simulink model "Glide_slope_controller_d"  (R2019b)
settings: Solver=VariableStepAuto  StartTime=0.0  StopTime=300  RelTol=1e-3
values from neighbouring files (symbols this model uses):
  A_gs = A_longitude_lo([1 3 4 2 5], [1 3 4 2 5])    [FindF16Dynamics.m]    (also in FindF16Dynamics_Chapter8.m)
  alpha = 8.49    [FindF16Dynamics.m]    (also in FindF16Dynamics_Chapter8.m = 10.4511; FindF16Dynamics_KIllian.m; trim_F16.m = alpha*pi/180)
  B_gs = A_longitude_lo([1 3 4 2 5], [6, 7])    [FindF16Dynamics.m]    (also in FindF16Dynamics_Chapter8.m)
  C_gs = C_longitude_lo([1 3 4 2 5], [1 3 4 2 5])    [FindF16Dynamics.m]    (also in FindF16Dynamics_Chapter8.m)
  D_gs = D_longitude_lo([1 3 4 2 5], [1])    [FindF16Dynamics.m]    (also in FindF16Dynamics_Chapter8.m = D_longitude_lo([1 3 4 2 5], [1, 2]))
  thrust = 5000    [FindF16Dynamics.m]    (also in FindF16Dynamics_Chapter8.m = 2826.8165; FindF16Dynamics_KIllian.m)
  velocity = 300    [FindF16Dynamics.m]    (also in FindF16Dynamics_Chapter8.m; FindF16Dynamics_KIllian.m = input('Enter the velocity for the simulation (ft/s):  '); FindF16Dynamics_Q6,7.m = 900; FindF16Dynamics_Q6-7.m = 900)
libraries: simulink x4
settings Model: Creator=tomas  LastModifiedBy=tomas

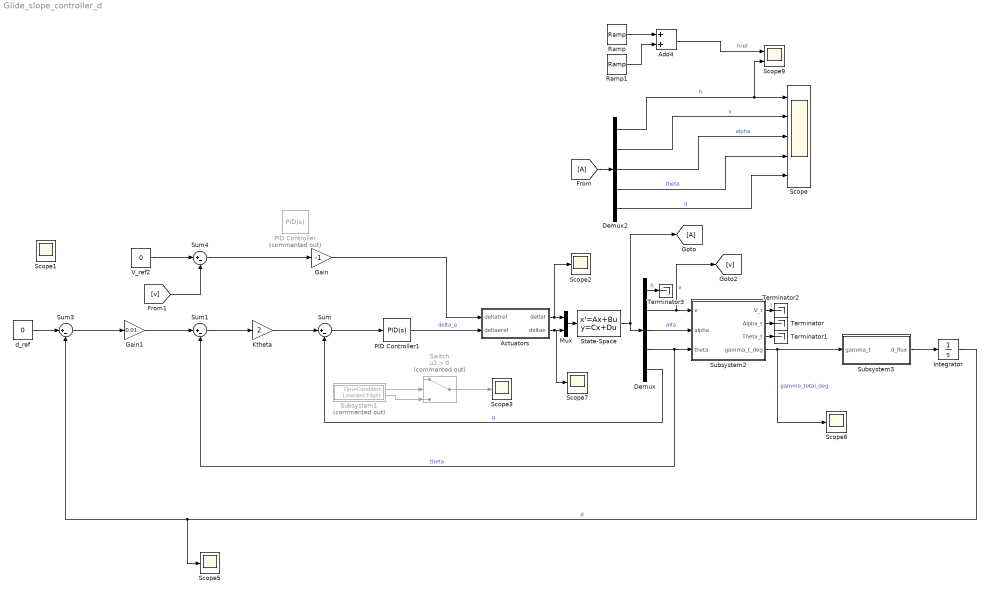
== system Glide_slope_controller_d ==
  Actuators : Subsystem
  Add4 : Sum
  Demux : Demux  Outputs=5
  Demux2 : Demux  Outputs=5
  Gain : Gain  Gain=-1
  Gain1 : Gain  Gain=0.01
  Integrator : Integrator
  Ktheta : Gain  Gain=2
  Mux : Mux  Inputs=2
  PID Controller : simulink/Continuous/PID Controller  Commented=on  Controller=PID  Form=Parallel  TimeDomain=Continuous-time  SampleTime=-1  IntegratorMethod=Forward Euler  FilterMethod=Forward Euler  ControllerParametersSource=internal  P=32442.6035152476  I=115590.834406017  D=865.549323517824  UseFilter=on  N=3789.88151864389  TunerSelectOption=Transfer Function Based (PID Tuner App)  InitialConditionSource=internal  InitialConditionForIntegrator=0  InitialConditionForFilter=0  DifferentiatorICPrevScaledInput=0  ExternalReset=none  TrackingMode=off  Kt=1  LimitOutput=off  UpperSaturationLimit=inf  LowerSaturationLimit=-inf  LinearizeAsGain=on  AntiWindupMode=none  Kb=1  POutMin=[]  POutMax=[]  IOutMin=[]  IOutMax=[]  DOutMin=[]  DOutMax=[]  NOutMin=[]  NOutMax=[]  SumOutMin=[]  SumOutMax=[]  SaturationOutMin=[]  SaturationOutMax=[]  PParamMin=[]  PParamMax=[]  IParamMin=[]  IParamMax=[]  DParamMin=[]  DParamMax=[]  NParamMin=[]  NParamMax=[]  KbParamMin=[]  KbParamMax=[]  KtParamMin=[]  KtParamMax=[]  KbOutMin=[]  KbOutMax=[]  KtOutMin=[]  KtOutMax=[]  IntegratorOutMin=[]  IntegratorOutMax=[]  FilterOutMin=[]  FilterOutMax=[]  SumI1OutMin=[]  SumI1OutMax=[]  SumI2OutMin=[]  SumI2OutMax=[]  SumI3OutMin=[]  SumI3OutMax=[]  SumI4OutMin=[]  SumI4OutMax=[]  SumDOutMin=[]  SumDOutMax=[]  DifferentiatorOutMin=[]  DifferentiatorOutMax=[]  FilterDiffOutCoefMin=[]  FilterDiffOutCoefMax=[]  ReciprocalOutMin=[]  ReciprocalOutMax=[]  SumDenOutMin=[]  SumDenOutMax=[]  SumNumOutMin=[]  SumNumOutMax=[]  DivideOutMin=[]  DivideOutMax=[]  IntegratorContinuousStateAttributes=''  IntegratorStateMustResolveToSignalObject=off  IntegratorRTWStateStorageClass=Auto  FilterContinuousStateAttributes=''  FilterStateMustResolveToSignalObject=off  FilterRTWStateStorageClass=Auto  ParallelPVariant=InternalParameters  IdealPVariant=Disabled  IVariant=InternalParameters  DVariant=InternalParameters  IntegratorVariant=Continuous  SatVariant=Disabled  AWVariant=Passthrough  PCopyVariant=Disabled  TRVariant=Disabled  FdbkBlocksVariant=Forward  IdealPFdbkVariant=Disabled  SatFdbkVariant=Disabled  DerivativeFilterVariant=ContFilter  NVariant=InternalParameters  NCopyVariant=Disabled  FilterICVariant=InternalICsFilter  IntegratorICVariant=InternalICs  ExternalResetVariant=Disabled  TRSumVariant=Passthrough  SumFdbkVariant=Disabled  SumVariant=Sum_PID
  PID Controller1 : simulink/Continuous/PID Controller  Controller=PID  Form=Parallel  TimeDomain=Continuous-time  SampleTime=-1  IntegratorMethod=Forward Euler  FilterMethod=Forward Euler  ControllerParametersSource=internal  P=-5  I=-1  D=-1  UseFilter=on  N=100  TunerSelectOption=Transfer Function Based (PID Tuner App)  InitialConditionSource=internal  InitialConditionForIntegrator=0  InitialConditionForFilter=0  DifferentiatorICPrevScaledInput=0  ExternalReset=none  TrackingMode=off  Kt=1  LimitOutput=off  UpperSaturationLimit=inf  LowerSaturationLimit=-inf  LinearizeAsGain=on  AntiWindupMode=none  Kb=1  POutMin=[]  POutMax=[]  IOutMin=[]  IOutMax=[]  DOutMin=[]  DOutMax=[]  NOutMin=[]  NOutMax=[]  SumOutMin=[]  SumOutMax=[]  SaturationOutMin=[]  SaturationOutMax=[]  PParamMin=[]  PParamMax=[]  IParamMin=[]  IParamMax=[]  DParamMin=[]  DParamMax=[]  NParamMin=[]  NParamMax=[]  KbParamMin=[]  KbParamMax=[]  KtParamMin=[]  KtParamMax=[]  KbOutMin=[]  KbOutMax=[]  KtOutMin=[]  KtOutMax=[]  IntegratorOutMin=[]  IntegratorOutMax=[]  FilterOutMin=[]  FilterOutMax=[]  SumI1OutMin=[]  SumI1OutMax=[]  SumI2OutMin=[]  SumI2OutMax=[]  SumI3OutMin=[]  SumI3OutMax=[]  SumI4OutMin=[]  SumI4OutMax=[]  SumDOutMin=[]  SumDOutMax=[]  DifferentiatorOutMin=[]  DifferentiatorOutMax=[]  FilterDiffOutCoefMin=[]  FilterDiffOutCoefMax=[]  ReciprocalOutMin=[]  ReciprocalOutMax=[]  SumDenOutMin=[]  SumDenOutMax=[]  SumNumOutMin=[]  SumNumOutMax=[]  DivideOutMin=[]  DivideOutMax=[]  IntegratorContinuousStateAttributes=''  IntegratorStateMustResolveToSignalObject=off  IntegratorRTWStateStorageClass=Auto  FilterContinuousStateAttributes=''  FilterStateMustResolveToSignalObject=off  FilterRTWStateStorageClass=Auto  ParallelPVariant=InternalParameters  IdealPVariant=Disabled  IVariant=InternalParameters  DVariant=InternalParameters  IntegratorVariant=Continuous  SatVariant=Disabled  AWVariant=Passthrough  PCopyVariant=Disabled  TRVariant=Disabled  FdbkBlocksVariant=Forward  IdealPFdbkVariant=Disabled  SatFdbkVariant=Disabled  DerivativeFilterVariant=ContFilter  NVariant=InternalParameters  NCopyVariant=Disabled  FilterICVariant=InternalICsFilter  IntegratorICVariant=InternalICs  ExternalResetVariant=Disabled  TRSumVariant=Passthrough  SumFdbkVariant=Disabled  SumVariant=Sum_PID
  Ramp : simulink/Sources/Ramp  slope=-5*pi  start=10  InitialOutput=0
  Ramp1 : simulink/Sources/Ramp  slope=5*pi  start=t_maneuver_1  InitialOutput=0
  Scope : Scope  NumInputPorts=5
  Scope{1..3,5..7} (6 alike) : Scope
  Scope9 : Scope  NumInputPorts=2
  State-Space : StateSpace  A=A_gs  B=B_gs  C=C_gs  D=D_gs  InitialCondition=0
  Subsystem1 : Subsystem  Commented=on
  Subsystem2 : Subsystem
  Subsystem3 : Subsystem
  Sum{,1,3..4} (4 alike) : Sum  Inputs=|+-
  Switch : Switch  Commented=on  Criteria=u2 > Threshold
  Terminator{,1..3} (4 alike) : Terminator
  V_ref2 : Constant  Value=0
  d_ref : Constant  Value=0
  wires:
  State-Space/1 -> Demux/1, [A]
  Demux/5 -> Sum/2  "q"
  [A] -> Demux2/1
  Demux2/1 -> Scope9/2, Scope/1  "h"
  Demux2/2 -> Scope/2  "v"
  Demux2/3 -> Scope/3  "alpha"
  Demux2/4 -> Scope/4  "theta"
  Demux2/5 -> Scope/5  "q"
  Sum1/1 -> Ktheta/1
  Sum/1 -> PID Controller1/1
  Subsystem2/4(gamma_t_deg) -> Scope6/1, Subsystem3/1(gamma_t)  "gamma_total_deg"
  Subsystem3/1(d_flux) -> Integrator/1
  Integrator/1 -> Sum3/2, Scope5/1  "d"
  Mux/1 -> State-Space/1
  Demux/4 -> Subsystem2/3(theta), Sum1/2  "theta"
  Actuators/2(deltae) -> Scope7/1, Mux/2
  Actuators/1(deltat) -> Mux/1, Scope2/1
  [v] -> Sum4/2
  V_ref2/1 -> Sum4/1
  Switch/1 -> Scope3/1
  Subsystem1/1(TimeCondition) -> Switch/2
  Subsystem1/2(Levelled Flight) -> Switch/3
  Ramp/1 -> Add4/1
  Ramp1/1 -> Add4/2
  Add4/1 -> Scope9/1  "href"
  Demux/3 -> Subsystem2/2(alpha)  "alfa"
  Demux/2 -> [v], Subsystem2/1(v)  "v"
  Subsystem2/2(Alpha_t) -> Terminator/1
  Subsystem2/3(Theta_t) -> Terminator1/1
  Ktheta/1 -> Sum/1
  Subsystem2/1(V_t) -> Terminator2/1  "l"
  Gain1/1 -> Sum1/1
  Sum3/1 -> Gain1/1
  Sum4/1 -> Gain/1
  Demux/1 -> Terminator3/1  "h"
  Gain/1 -> Actuators/1(deltatref)
  PID Controller1/1 -> Actuators/2("deltaeref ")  "delta_e"
  d_ref/1 -> Sum3/1

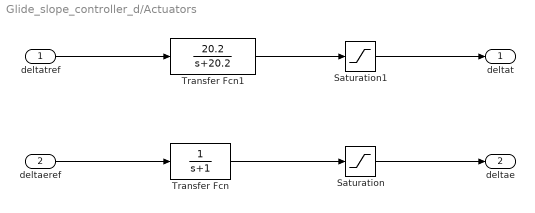
== system Glide_slope_controller_d/Actuators ==
  deltatref : Inport
  "deltaeref " : Inport  Port=2
  Saturation : Saturate  UpperLimit=14.5489  LowerLimit=-35.4511
  Saturation1 : Saturate  UpperLimit=19000-thrust  LowerLimit=1000-thrust
  Transfer Fcn : TransferFcn  Denominator=[1 1]
  Transfer Fcn1 : TransferFcn  Numerator=[20.2]  Denominator=[1 20.2]
  deltat : Outport
  deltae : Outport  Port=2
  wires:
  "deltaeref "/1 -> Transfer Fcn/1
  Transfer Fcn/1 -> Saturation/1
  Saturation/1 -> deltae/1
  Saturation1/1 -> deltat/1
  Transfer Fcn1/1 -> Saturation1/1
  deltatref/1 -> Transfer Fcn1/1

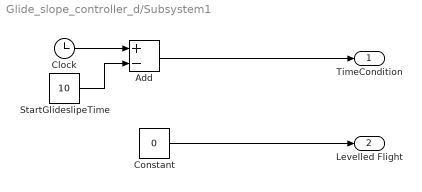
== system Glide_slope_controller_d/Subsystem1 ==
  Add : Sum  Inputs=+-
  Clock : Clock
  Constant : Constant  Value=0
  StartGlideslipeTime : Constant  Value=10
  TimeCondition : Outport
  Levelled Flight : Outport  Port=2
  wires:
  Clock/1 -> Add/1
  StartGlideslipeTime/1 -> Add/2
  Add/1 -> TimeCondition/1
  Constant/1 -> Levelled Flight/1

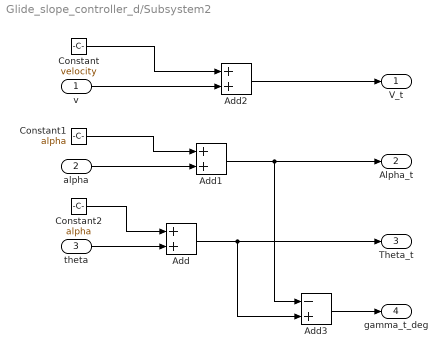
== system Glide_slope_controller_d/Subsystem2 ==
  v : Inport
  alpha : Inport  Port=2
  theta : Inport  Port=3
  Add : Sum
  Add1 : Sum
  Add2 : Sum
  Add3 : Sum  Inputs=-+
  Constant : Constant  Value=velocity
  Constant1 : Constant  Value=alpha
  Constant2 : Constant  Value=alpha
  V_t : Outport
  Alpha_t : Outport  Port=2
  Theta_t : Outport  Port=3
  gamma_t_deg : Outport  Port=4
  wires:
  Constant2/1 -> Add/1
  theta/1 -> Add/2
  Add/1 -> Theta_t/1, Add3/2
  Constant/1 -> Add2/1
  v/1 -> Add2/2
  Add2/1 -> V_t/1
  alpha/1 -> Add1/2
  Constant1/1 -> Add1/1
  Add1/1 -> Alpha_t/1, Add3/1
  Add3/1 -> gamma_t_deg/1

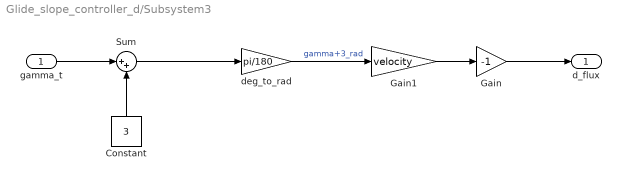
== system Glide_slope_controller_d/Subsystem3 ==
  gamma_t : Inport
  Constant : Constant  Value=3
  Gain : Gain  Gain=-1
  Gain1 : Gain  Gain=velocity
  Sum : Sum  Inputs=|++
  deg_to_rad : Gain  Gain=pi/180
  d_flux : Outport
  wires:
  deg_to_rad/1 -> Gain1/1  "gamma+3_rad"
  gamma_t/1 -> Sum/1
  Constant/1 -> Sum/2
  Sum/1 -> deg_to_rad/1
  Gain1/1 -> Gain/1
  Gain/1 -> d_flux/1
